simulink model "chap5_1sim"  (Simulink 7.0)
settings: Solver=ode45  StartTime=0.0  StopTime=30  RelTol=1e-5
settings Model: Creator=hp  LastModifiedBy=eleliuj  ExtModeTrigMode=oneshot  ExtModeArmWhenConnect=off
settings DataIOCC: LimitDataPoints=off  SignalLoggingName=sigsOut
settings OptimizationCC: BooleanDataType=off
settings DebuggingCC: SaveWithParameterizedLinksMsg=none  SignalResolutionControl=TryResolveAllWithWarning  SolverPrmCheckMsg=none  MultiTaskDSMMsg=warning  MultiTaskCondExecSysMsg=none  StrictBusMsg=None
settings HardwareCC: TargetUnknown=on
settings RTWCC: IncludeERTFirstTime=on
settings GRTTargetCC: TargetFcnLib=ansi_tfl_tmw.mat

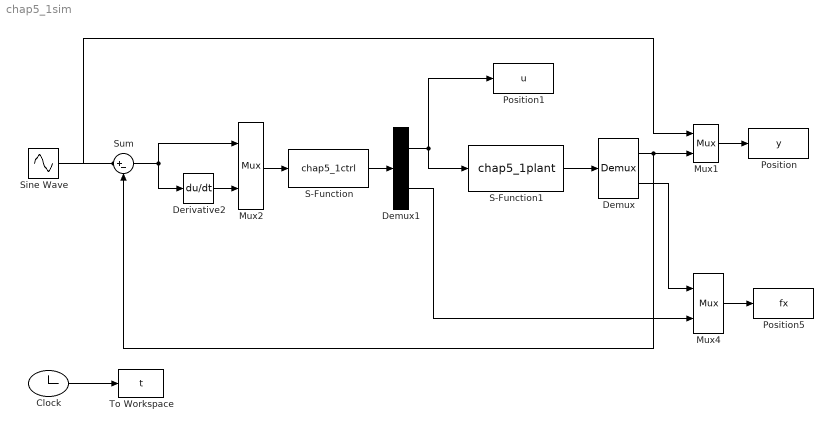
== system chap5_1sim ==
  Clock : Clock
      settings: Decimation=10
  Demux : Demux  Outputs=2
  Demux1 : Demux  Outputs=2
  Derivative2 : Derivative
  Mux1 : Mux  Inputs=2
  Mux2 : Mux  Inputs=2
  Mux4 : Mux  Inputs=2
  Position : ToWorkspace  VariableName=y  SampleTime=-1  SaveFormat=Array
  Position1 : ToWorkspace  VariableName=u  SampleTime=-1  SaveFormat=Array
  Position5 : ToWorkspace  VariableName=fx  SampleTime=-1  SaveFormat=Array
  S-Function : S-Function  FunctionName=chap5_1ctrl
  S-Function1 : S-Function  FunctionName=chap5_1plant
  Sine Wave : Sin  Amplitude=0.1  SampleTime=0
  Sum : Sum  Inputs=|+-  OutDataType=sfix(16)  OutScaling=2^0  SaturateOnIntegerOverflow=on
  To Workspace : ToWorkspace  VariableName=t  SampleTime=-1  SaveFormat=Array
  wires:
  Mux1/1 -> Position/1
  Demux/1 -> Mux1/2, Sum/2
  S-Function1/1 -> Demux/1
  S-Function/1 -> Demux1/1
  Clock/1 -> To Workspace/1
  Mux4/1 -> Position5/1
  Demux/2 -> Mux4/1
  Demux1/1 -> S-Function1/1, Position1/1
  Demux1/2 -> Mux4/2
  Sine Wave/1 -> Mux1/1, Sum/1
  Mux2/1 -> S-Function/1
  Sum/1 -> Mux2/1, Derivative2/1
  Derivative2/1 -> Mux2/2
